simulink model "rtwdemo_typeconveml"  (Simulink 7.1)
settings: Solver=FixedStepDiscrete  StartTime=0.0  StopTime=10.0  RelTol=1e-3
settings Model: Creator=ajayaram  LastModifiedBy=ajayaram
settings OptimizationCC: InlineParams=on  OptimizeModelRefInitCode=on  LifeSpan=1
settings RTWCC: SystemTargetFile=ert.tlc  GenCodeOnly=on  GenerateMakefile=off  TemplateMakefile=ert_default_tmf  Description=Real-Time Workshop Embedded Coder (no auto configuration)  GenerateReport=on  ProcessScript=ert_make_rtw_hook  IncludeHyperlinkInReport=on  LaunchReport=on
settings CodeAppCC: GenerateComments=off  IgnoreCustomStorageClasses=off  SimulinkBlockComments=off
settings ERTTargetCC: GenerateSampleERTMain=on  InlinedParameterPlacement=NonHierarchical  ERTCustomFileTemplate=example_file_process.tlc

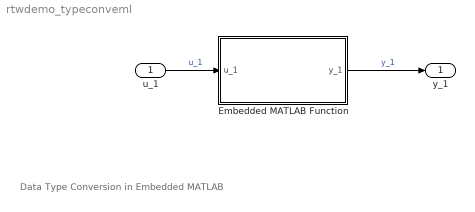
== system rtwdemo_typeconveml ==
  note: Data Type Conversion in Embedded MATLAB
  u_1 : Inport  DataType=int32  OutDataType=sfix(16)  OutScaling=2^0  OutDataTypeStr=int32
  Embedded MATLAB Function : Stateflow chart
  y_1 : Outport  OutDataType=sfix(16)  OutScaling=2^0
  wires:
  u_1/1 -> Embedded MATLAB Function/1(u_1)  "u_1"
  Embedded MATLAB Function/1(y_1) -> y_1/1  "y_1"

== matlab function Embedded MATLAB Function ==
  data: u_1 input double; y_1 output double
function y_1 = typeconv(u_1)

y_1 = double(u_1);

% NOTE: 'single' data type corresponds to 32-bit floating point
